simulink model "dong_hoc_thuan"  (R2016a)
settings: Solver=VariableStepAuto  StartTime=0.0  StopTime=10.0  RelTol=1e-3
settings Model: Creator=admin  LastModifiedBy=admin

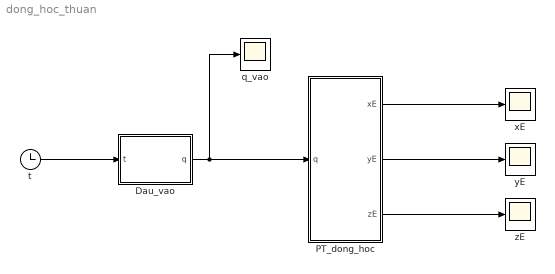
== system dong_hoc_thuan ==
  Dau_vao : MATLAB Function  TreatAsAtomicUnit=on
  PT_dong_hoc : MATLAB Function  TreatAsAtomicUnit=on
  q_vao : Scope
  "t " : Clock
  xE : Scope
  yE : Scope
  zE : Scope
  wires:
  "t "/1 -> Dau_vao/1(t)
  Dau_vao/1(q) -> q_vao/1, PT_dong_hoc/1(q)
  PT_dong_hoc/1(xE) -> xE/1
  PT_dong_hoc/2(yE) -> yE/1
  PT_dong_hoc/3(zE) -> zE/1

== matlab function dong_hoc_thuan/PT_dong_hoc ==
  data: q input; xE output; yE output; zE output
function [xE,yE,zE] = fcn(q)
[l1,l2,l3,l4,l5] = Parameter();
%PT diem cuoi xE,yE,zE
xE = -sin(q(3,1)) * cos(q(4,1)) * cos(q(1,1)) * q(5,1) - sin(q(1,1)) * sin(q(4,1)) * q(5,1) + cos(q(1,1)) * cos(q(3,1)) * l4 + cos(q(1,1)) * l3 * cos(q(3,1)) + cos(q(1,1)) * q(2,1);
yE = -sin(q(3,1)) * sin(q(1,1)) * cos(q(4,1)) * q(5,1) + sin(q(4,1)) * cos(q(1,1)) * q(5,1) + sin(q(1,1)) * cos(q(3,1)) * l4 + sin(q(1,1)) * l3 * cos(q(3,1)) + sin(q(1,1)) * q(2,1);
zE = -cos(q(3,1)) * cos(q(4,1)) * q(5,1) - sin(q(3,1)) * l4 - l3 * sin(q(3,1)) + l1;
end

== matlab function dong_hoc_thuan/Dau_vao ==
  data: t input; q output
function q = fcn(t)
%dau vao khai bao cac bien khop
q=zeros(5,1);
q(1,1)=0.5*sin(t+pi/3);
q(2,1)=0.42*sin(t);
q(3,1)=cos(t);
q(4,1)=sin((pi/2)*t);
q(5,1)=0.47*cos(t);
end
